simulink model "sim_pil_test"  (Simulink 8.1)
settings: Solver=FixedStepDiscrete  StartTime=0.0  StopTime=100.0  FixedStep=T  RelTol=1e-3
PostLoadFcn:
  | sim_test_data
StartFcn:
  | sim_test_data
values from neighbouring files (symbols this model uses):
  T = 1    [sim_test_data.m]
settings Model: Creator=evarshavskaya  LastModifiedBy=evarshavskaya
settings DataIOCC: ExternalInput=off  InitialState=off  LimitDataPoints=off  SaveOutput=off  SignalLogging=off  SaveTime=off
settings OptimizationCC: InlineParams=on  OptimizeModelRefInitCode=on  LifeSpan=1
settings DebuggingCC: InheritedTsInSrcMsg=none  SingleTaskRateTransMsg=error  UnconnectedInputMsg=error  UnconnectedOutputMsg=error  UnconnectedLineMsg=error  UnknownTsInhSupMsg=error
settings HardwareCC: ProdLargestAtomicInteger=Long  ProdLargestAtomicFloat=Double  ProdIntDivRoundTo=Zero  ProdEndianess=BigEndian  ProdHWDeviceType=Freescale->32-bit PowerPC
settings RTWCC: SystemTargetFile=rappid564xl.tlc  MakeCommand=rappid_564xl_make_rtw  TemplateMakefile=rappid_564xl_default_tmf  PostCodeGenCommand=rappid_analyzegencode(buildInfo)  Description=RAppID Toolbox MPC564xL Code Generation Target (rappid)  ProcessScript=rappid564xl_make_rtw_hook
settings CodeAppCC: IgnoreCustomStorageClasses=off  MaxIdLength=63  CustomSymbolStrType=$N$R$M  InternalIdentifier=Classic
settings STFCustomTargetCC: CodeReplacementLibrary=ANSI_C  GenerateSampleERTMain=on  ModelReferenceCompliant=off  CombineOutputUpdateFcns=on  ERTCustomFileBanners=on  SupportContinuousTime=off  SupportNonInlinedSFcns=off  MATLABClassNameForMDSCustomization=Simulink.SoftwareTarget.ERTCustomization  GRTInterface=off  SystemTargetFile=rappid564xl.tlc
settings ERTTargetCC: CodeReplacementLibrary=ANSI_C  MultiwordLength=2048  GenerateSampleERTMain=on  ModelReferenceCompliant=off  ParMdlRefBuildCompliant=off  CompOptLevelCompliant=off  ConcurrentExecutionCompliant=off  ERTFirstTimeCompliant=off  ModelStepFunctionPrototypeControlCompliant=off  CPPClassGenCompliant=off  ExtModeMexFile=noextcomm  InlinedParameterPlacement=NonHierarchical  ERTCustomFileTemplate=example_file_process.tlc  ConvertIfToSwitch=off  SuppressUnreachableDefaultCases=off

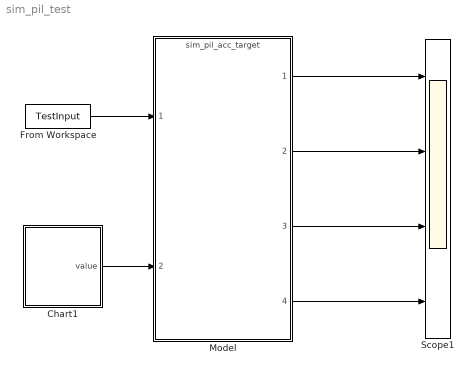
== system sim_pil_test ==
  Chart1 : Stateflow chart  TreatAsAtomicUnit=on
  From Workspace : FromWorkspace  VariableName=TestInput  SampleTime=T
  Model : ModelReference  ModelNameDialog=sim_pil_acc_target  SimulationMode=Processor-in-the-loop (PIL)  ModelReferenceVersion=1.162  CopyOfModelName=sim_pil_acc_target  DefaultDataLogging=off
  Scope1 : Scope  NumInputPorts=4
      settings: TimeRange=100  YMin=5000~-1~1250~0  YMax=30000~1~1290~1
  wires:
  From Workspace/1 -> Model/1
  Model/1 -> Scope1/1
  Model/2 -> Scope1/2
  Model/3 -> Scope1/3
  Model/4 -> Scope1/4
  Chart1/1(value) -> Model/2

== stateflow chart Chart1 ==
  settings: executeAtInitialization=1
  state A
    du:
    cntr=cntr+0.2;
    value=cntr;
    ex:
    cntr = -3.14;
  (default) -> A : {cntr=0;}
  A -> A : [cntr >= 3.14]
  data: cntr local single =0; value output single
